simulink model "gm_gauss_sobel_rgb_64bit_full"  (R2022a)
settings: Solver=VariableStepAuto  StartTime=0.0  StopTime=10.0  RelTol=1e-3
undefined symbols (not defined in the file or in its folder): blueMax, blueMin, gray, greenMax, greenMin, redMax, redMin
libraries: hdlsllib x62, visionhdlio x6, visionsources x2
(part 2 of 3)

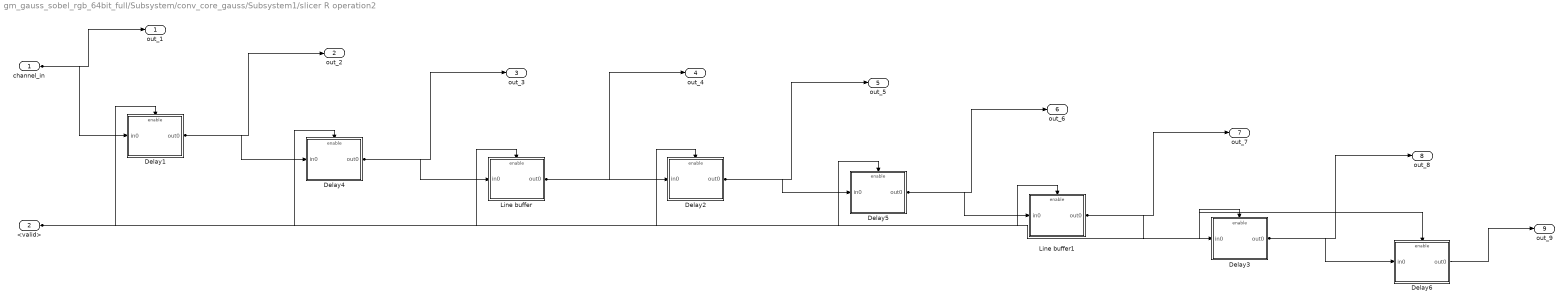
== system gm_gauss_sobel_rgb_64bit_full/Subsystem/conv_core_gauss/Subsystem1/slicer R operation2 ==
  channel_in : Inport  OutDataTypeStr=uint8  PortDimensions=1  SampleTime=2.77039007092199e-06
  <valid> : Inport  Port=2  OutDataTypeStr=boolean  SampleTime=2.77039007092199e-06
  Delay1 : Subsystem
      settings: MinAlgLoopOccurrences=on
  Delay2 : Subsystem
      settings: MinAlgLoopOccurrences=on
  Delay3 : Subsystem
      settings: MinAlgLoopOccurrences=on
  Delay4 : Subsystem
      settings: MinAlgLoopOccurrences=on
  Delay5 : Subsystem
      settings: MinAlgLoopOccurrences=on
  Delay6 : Subsystem
      settings: MinAlgLoopOccurrences=on
  Line buffer : Subsystem
      settings: MinAlgLoopOccurrences=on
  Line buffer1 : Subsystem
      settings: MinAlgLoopOccurrences=on
  out_1 : Outport  SampleTime=2.77039007092199e-06  InitialOutput=0  VectorParamsAs1DForOutWhenUnconnected=off
  out_2 : Outport  Port=2  SampleTime=2.77039007092199e-06  InitialOutput=0  VectorParamsAs1DForOutWhenUnconnected=off
  out_3 : Outport  Port=3  SampleTime=2.77039007092199e-06  InitialOutput=0  VectorParamsAs1DForOutWhenUnconnected=off
  out_4 : Outport  Port=4  SampleTime=2.77039007092199e-06  InitialOutput=0  VectorParamsAs1DForOutWhenUnconnected=off
  out_5 : Outport  Port=5  SampleTime=2.77039007092199e-06  InitialOutput=0  VectorParamsAs1DForOutWhenUnconnected=off
  out_6 : Outport  Port=6  SampleTime=2.77039007092199e-06  InitialOutput=0  VectorParamsAs1DForOutWhenUnconnected=off
  out_7 : Outport  Port=7  SampleTime=2.77039007092199e-06  InitialOutput=0  VectorParamsAs1DForOutWhenUnconnected=off
  out_8 : Outport  Port=8  SampleTime=2.77039007092199e-06  InitialOutput=0  VectorParamsAs1DForOutWhenUnconnected=off
  out_9 : Outport  Port=9  SampleTime=2.77039007092199e-06  InitialOutput=0  VectorParamsAs1DForOutWhenUnconnected=off
  wires:
  channel_in/1 -> Delay1/1(in0), out_1/1
  Delay1/1(out0) -> Delay4/1(in0), out_2/1
  Delay2/1(out0) -> Delay5/1(in0), out_5/1
  Delay3/1(out0) -> Delay6/1(in0), out_8/1
  Delay4/1(out0) -> Line buffer/1(in0), out_3/1
  Delay5/1(out0) -> Line buffer1/1(in0), out_6/1
  Delay6/1(out0) -> out_9/1
  Line buffer/1(out0) -> Delay2/1(in0), out_4/1
  Line buffer1/1(out0) -> Delay3/1(in0), out_7/1
  <valid>/1 -> Line buffer1/Enable, Line buffer/Enable, Delay6/Enable, Delay5/Enable, Delay4/Enable, Delay3/Enable, Delay2/Enable, Delay1/Enable

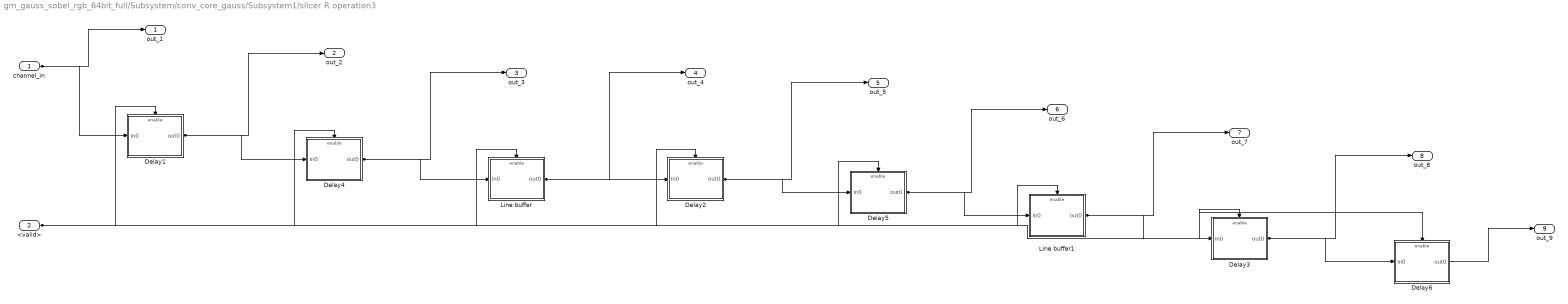
== system gm_gauss_sobel_rgb_64bit_full/Subsystem/conv_core_gauss/Subsystem1/slicer R operation3 ==
  channel_in : Inport  OutDataTypeStr=uint8  PortDimensions=1  SampleTime=2.77039007092199e-06
  <valid> : Inport  Port=2  OutDataTypeStr=boolean  SampleTime=2.77039007092199e-06
  Delay1 : Subsystem
      settings: MinAlgLoopOccurrences=on
  Delay2 : Subsystem
      settings: MinAlgLoopOccurrences=on
  Delay3 : Subsystem
      settings: MinAlgLoopOccurrences=on
  Delay4 : Subsystem
      settings: MinAlgLoopOccurrences=on
  Delay5 : Subsystem
      settings: MinAlgLoopOccurrences=on
  Delay6 : Subsystem
      settings: MinAlgLoopOccurrences=on
  Line buffer : Subsystem
      settings: MinAlgLoopOccurrences=on
  Line buffer1 : Subsystem
      settings: MinAlgLoopOccurrences=on
  out_1 : Outport  SampleTime=2.77039007092199e-06  InitialOutput=0  VectorParamsAs1DForOutWhenUnconnected=off
  out_2 : Outport  Port=2  SampleTime=2.77039007092199e-06  InitialOutput=0  VectorParamsAs1DForOutWhenUnconnected=off
  out_3 : Outport  Port=3  SampleTime=2.77039007092199e-06  InitialOutput=0  VectorParamsAs1DForOutWhenUnconnected=off
  out_4 : Outport  Port=4  SampleTime=2.77039007092199e-06  InitialOutput=0  VectorParamsAs1DForOutWhenUnconnected=off
  out_5 : Outport  Port=5  SampleTime=2.77039007092199e-06  InitialOutput=0  VectorParamsAs1DForOutWhenUnconnected=off
  out_6 : Outport  Port=6  SampleTime=2.77039007092199e-06  InitialOutput=0  VectorParamsAs1DForOutWhenUnconnected=off
  out_7 : Outport  Port=7  SampleTime=2.77039007092199e-06  InitialOutput=0  VectorParamsAs1DForOutWhenUnconnected=off
  out_8 : Outport  Port=8  SampleTime=2.77039007092199e-06  InitialOutput=0  VectorParamsAs1DForOutWhenUnconnected=off
  out_9 : Outport  Port=9  SampleTime=2.77039007092199e-06  InitialOutput=0  VectorParamsAs1DForOutWhenUnconnected=off
  wires:
  channel_in/1 -> Delay1/1(in0), out_1/1
  Delay1/1(out0) -> Delay4/1(in0), out_2/1
  Delay2/1(out0) -> Delay5/1(in0), out_5/1
  Delay3/1(out0) -> Delay6/1(in0), out_8/1
  Delay4/1(out0) -> Line buffer/1(in0), out_3/1
  Delay5/1(out0) -> Line buffer1/1(in0), out_6/1
  Delay6/1(out0) -> out_9/1
  Line buffer/1(out0) -> Delay2/1(in0), out_4/1
  Line buffer1/1(out0) -> Delay3/1(in0), out_7/1
  <valid>/1 -> Line buffer1/Enable, Line buffer/Enable, Delay6/Enable, Delay5/Enable, Delay4/Enable, Delay3/Enable, Delay2/Enable, Delay1/Enable

== system gm_gauss_sobel_rgb_64bit_full/Subsystem/conv_core_gauss/Subsystem1/slicer R operation4 ==
  channel_in : Inport  OutDataTypeStr=uint8  PortDimensions=1  SampleTime=2.77039007092199e-06
  <valid> : Inport  Port=2  OutDataTypeStr=boolean  SampleTime=2.77039007092199e-06
  Delay1 : Subsystem
      settings: MinAlgLoopOccurrences=on
  Delay2 : Subsystem
      settings: MinAlgLoopOccurrences=on
  Delay3 : Subsystem
      settings: MinAlgLoopOccurrences=on
  Delay4 : Subsystem
      settings: MinAlgLoopOccurrences=on
  Delay5 : Subsystem
      settings: MinAlgLoopOccurrences=on
  Delay6 : Subsystem
      settings: MinAlgLoopOccurrences=on
  Line buffer : Subsystem
      settings: MinAlgLoopOccurrences=on
  Line buffer1 : Subsystem
      settings: MinAlgLoopOccurrences=on
  out_1 : Outport  SampleTime=2.77039007092199e-06  InitialOutput=0  VectorParamsAs1DForOutWhenUnconnected=off
  out_2 : Outport  Port=2  SampleTime=2.77039007092199e-06  InitialOutput=0  VectorParamsAs1DForOutWhenUnconnected=off
  out_3 : Outport  Port=3  SampleTime=2.77039007092199e-06  InitialOutput=0  VectorParamsAs1DForOutWhenUnconnected=off
  out_4 : Outport  Port=4  SampleTime=2.77039007092199e-06  InitialOutput=0  VectorParamsAs1DForOutWhenUnconnected=off
  out_5 : Outport  Port=5  SampleTime=2.77039007092199e-06  InitialOutput=0  VectorParamsAs1DForOutWhenUnconnected=off
  out_6 : Outport  Port=6  SampleTime=2.77039007092199e-06  InitialOutput=0  VectorParamsAs1DForOutWhenUnconnected=off
  out_7 : Outport  Port=7  SampleTime=2.77039007092199e-06  InitialOutput=0  VectorParamsAs1DForOutWhenUnconnected=off
  out_8 : Outport  Port=8  SampleTime=2.77039007092199e-06  InitialOutput=0  VectorParamsAs1DForOutWhenUnconnected=off
  out_9 : Outport  Port=9  SampleTime=2.77039007092199e-06  InitialOutput=0  VectorParamsAs1DForOutWhenUnconnected=off
  wires:
  channel_in/1 -> Delay1/1(in0), out_1/1
  Delay1/1(out0) -> Delay4/1(in0), out_2/1
  Delay2/1(out0) -> Delay5/1(in0), out_5/1
  Delay3/1(out0) -> Delay6/1(in0), out_8/1
  Delay4/1(out0) -> Line buffer/1(in0), out_3/1
  Delay5/1(out0) -> Line buffer1/1(in0), out_6/1
  Delay6/1(out0) -> out_9/1
  Line buffer/1(out0) -> Delay2/1(in0), out_4/1
  Line buffer1/1(out0) -> Delay3/1(in0), out_7/1
  <valid>/1 -> Line buffer1/Enable, Line buffer/Enable, Delay6/Enable, Delay5/Enable, Delay4/Enable, Delay3/Enable, Delay2/Enable, Delay1/Enable

== system gm_gauss_sobel_rgb_64bit_full/Subsystem/conv_core_gauss/Subsystem1/slicer R operation5 ==
  channel_in : Inport  OutDataTypeStr=uint8  PortDimensions=1  SampleTime=2.77039007092199e-06
  <valid> : Inport  Port=2  OutDataTypeStr=boolean  SampleTime=2.77039007092199e-06
  Delay1 : Subsystem
      settings: MinAlgLoopOccurrences=on
  Delay2 : Subsystem
      settings: MinAlgLoopOccurrences=on
  Delay3 : Subsystem
      settings: MinAlgLoopOccurrences=on
  Delay4 : Subsystem
      settings: MinAlgLoopOccurrences=on
  Delay5 : Subsystem
      settings: MinAlgLoopOccurrences=on
  Delay6 : Subsystem
      settings: MinAlgLoopOccurrences=on
  Line buffer : Subsystem
      settings: MinAlgLoopOccurrences=on
  Line buffer1 : Subsystem
      settings: MinAlgLoopOccurrences=on
  out_1 : Outport  SampleTime=2.77039007092199e-06  InitialOutput=0  VectorParamsAs1DForOutWhenUnconnected=off
  out_2 : Outport  Port=2  SampleTime=2.77039007092199e-06  InitialOutput=0  VectorParamsAs1DForOutWhenUnconnected=off
  out_3 : Outport  Port=3  SampleTime=2.77039007092199e-06  InitialOutput=0  VectorParamsAs1DForOutWhenUnconnected=off
  out_4 : Outport  Port=4  SampleTime=2.77039007092199e-06  InitialOutput=0  VectorParamsAs1DForOutWhenUnconnected=off
  out_5 : Outport  Port=5  SampleTime=2.77039007092199e-06  InitialOutput=0  VectorParamsAs1DForOutWhenUnconnected=off
  out_6 : Outport  Port=6  SampleTime=2.77039007092199e-06  InitialOutput=0  VectorParamsAs1DForOutWhenUnconnected=off
  out_7 : Outport  Port=7  SampleTime=2.77039007092199e-06  InitialOutput=0  VectorParamsAs1DForOutWhenUnconnected=off
  out_8 : Outport  Port=8  SampleTime=2.77039007092199e-06  InitialOutput=0  VectorParamsAs1DForOutWhenUnconnected=off
  out_9 : Outport  Port=9  SampleTime=2.77039007092199e-06  InitialOutput=0  VectorParamsAs1DForOutWhenUnconnected=off
  wires:
  channel_in/1 -> Delay1/1(in0), out_1/1
  Delay1/1(out0) -> Delay4/1(in0), out_2/1
  Delay2/1(out0) -> Delay5/1(in0), out_5/1
  Delay3/1(out0) -> Delay6/1(in0), out_8/1
  Delay4/1(out0) -> Line buffer/1(in0), out_3/1
  Delay5/1(out0) -> Line buffer1/1(in0), out_6/1
  Delay6/1(out0) -> out_9/1
  Line buffer/1(out0) -> Delay2/1(in0), out_4/1
  Line buffer1/1(out0) -> Delay3/1(in0), out_7/1
  <valid>/1 -> Line buffer1/Enable, Line buffer/Enable, Delay6/Enable, Delay5/Enable, Delay4/Enable, Delay3/Enable, Delay2/Enable, Delay1/Enable

== system gm_gauss_sobel_rgb_64bit_full/Subsystem/conv_core_gauss/Subsystem1/slicer R operation6 ==
  channel_in : Inport  OutDataTypeStr=uint8  PortDimensions=1  SampleTime=2.77039007092199e-06
  <valid> : Inport  Port=2  OutDataTypeStr=boolean  SampleTime=2.77039007092199e-06
  Delay1 : Subsystem
      settings: MinAlgLoopOccurrences=on
  Delay2 : Subsystem
      settings: MinAlgLoopOccurrences=on
  Delay3 : Subsystem
      settings: MinAlgLoopOccurrences=on
  Delay4 : Subsystem
      settings: MinAlgLoopOccurrences=on
  Delay5 : Subsystem
      settings: MinAlgLoopOccurrences=on
  Delay6 : Subsystem
      settings: MinAlgLoopOccurrences=on
  Line buffer : Subsystem
      settings: MinAlgLoopOccurrences=on
  Line buffer1 : Subsystem
      settings: MinAlgLoopOccurrences=on
  out_1 : Outport  SampleTime=2.77039007092199e-06  InitialOutput=0  VectorParamsAs1DForOutWhenUnconnected=off
  out_2 : Outport  Port=2  SampleTime=2.77039007092199e-06  InitialOutput=0  VectorParamsAs1DForOutWhenUnconnected=off
  out_3 : Outport  Port=3  SampleTime=2.77039007092199e-06  InitialOutput=0  VectorParamsAs1DForOutWhenUnconnected=off
  out_4 : Outport  Port=4  SampleTime=2.77039007092199e-06  InitialOutput=0  VectorParamsAs1DForOutWhenUnconnected=off
  out_5 : Outport  Port=5  SampleTime=2.77039007092199e-06  InitialOutput=0  VectorParamsAs1DForOutWhenUnconnected=off
  out_6 : Outport  Port=6  SampleTime=2.77039007092199e-06  InitialOutput=0  VectorParamsAs1DForOutWhenUnconnected=off
  out_7 : Outport  Port=7  SampleTime=2.77039007092199e-06  InitialOutput=0  VectorParamsAs1DForOutWhenUnconnected=off
  out_8 : Outport  Port=8  SampleTime=2.77039007092199e-06  InitialOutput=0  VectorParamsAs1DForOutWhenUnconnected=off
  out_9 : Outport  Port=9  SampleTime=2.77039007092199e-06  InitialOutput=0  VectorParamsAs1DForOutWhenUnconnected=off
  wires:
  channel_in/1 -> Delay1/1(in0), out_1/1
  Delay1/1(out0) -> Delay4/1(in0), out_2/1
  Delay2/1(out0) -> Delay5/1(in0), out_5/1
  Delay3/1(out0) -> Delay6/1(in0), out_8/1
  Delay4/1(out0) -> Line buffer/1(in0), out_3/1
  Delay5/1(out0) -> Line buffer1/1(in0), out_6/1
  Delay6/1(out0) -> out_9/1
  Line buffer/1(out0) -> Delay2/1(in0), out_4/1
  Line buffer1/1(out0) -> Delay3/1(in0), out_7/1
  <valid>/1 -> Line buffer1/Enable, Line buffer/Enable, Delay6/Enable, Delay5/Enable, Delay4/Enable, Delay3/Enable, Delay2/Enable, Delay1/Enable

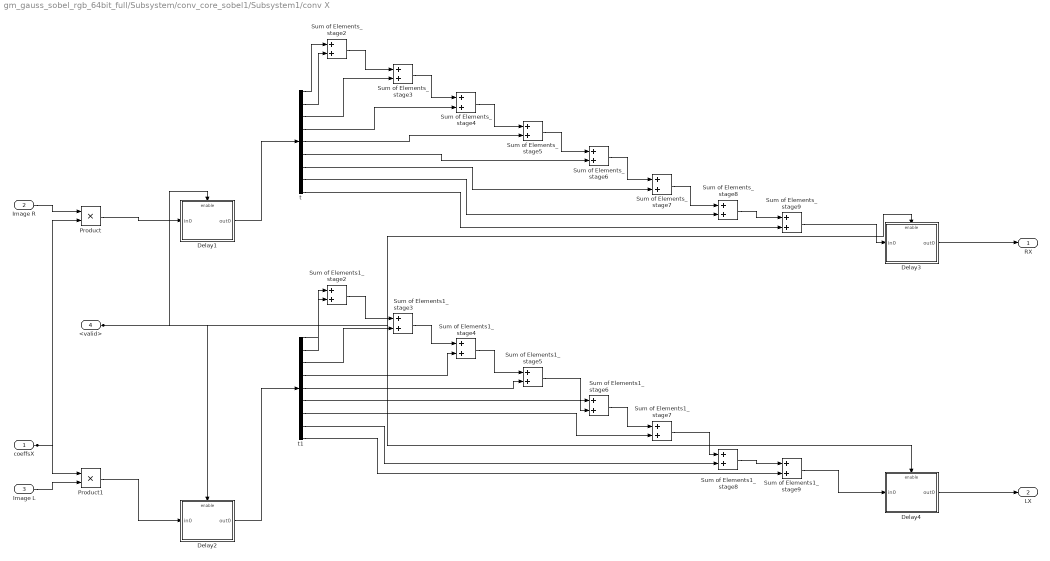
== system gm_gauss_sobel_rgb_64bit_full/Subsystem/conv_core_sobel1/Subsystem1/conv X ==
  coeffsX : Inport  OutDataTypeStr=int8  PortDimensions=[9]  SampleTime=2.77039007092199e-06
  Image R : Inport  Port=2  OutDataTypeStr=uint8  PortDimensions=[9]  SampleTime=2.77039007092199e-06
  Image L : Inport  Port=3  OutDataTypeStr=uint8  PortDimensions=[9]  SampleTime=2.77039007092199e-06
  <valid> : Inport  Port=4  OutDataTypeStr=boolean  SampleTime=2.77039007092199e-06
  Delay1 : Subsystem
      settings: MinAlgLoopOccurrences=on
  Delay2 : Subsystem
      settings: MinAlgLoopOccurrences=on
  Delay3 : Subsystem
      settings: MinAlgLoopOccurrences=on
  Delay4 : Subsystem
      settings: MinAlgLoopOccurrences=on
  Product : Product  Inputs=**  OutDataTypeStr=int16  SaturateOnIntegerOverflow=on  SampleTime=2.77039007092199e-06
  Product1 : Product  Inputs=**  OutDataTypeStr=int16  SaturateOnIntegerOverflow=on  SampleTime=2.77039007092199e-06
  Sum of Elements1_stage{2..8} (7 alike) : Sum  AccumDataTypeStr=int32  OutDataTypeStr=int32  SaturateOnIntegerOverflow=on  SampleTime=2.77039007092199e-06
  Sum of Elements1_stage9 : Sum  AccumDataTypeStr=int32  OutDataTypeStr=uint8  SaturateOnIntegerOverflow=on  SampleTime=2.77039007092199e-06
  Sum of Elements_stage{2..8} (7 alike) : Sum  AccumDataTypeStr=int32  OutDataTypeStr=int32  SaturateOnIntegerOverflow=on  SampleTime=2.77039007092199e-06
  Sum of Elements_stage9 : Sum  AccumDataTypeStr=int32  OutDataTypeStr=uint8  SaturateOnIntegerOverflow=on  SampleTime=2.77039007092199e-06
  t : Demux  Outputs=9
  t1 : Demux  Outputs=9
  RX : Outport  SampleTime=2.77039007092199e-06  InitialOutput=0
  LX : Outport  Port=2  SampleTime=2.77039007092199e-06  InitialOutput=0
  wires:
  coeffsX/1 -> Product1/1, Product/2
  Image R/1 -> Product/1
  Image L/1 -> Product1/2
  Delay1/1(out0) -> t/1
  Delay2/1(out0) -> t1/1
  Delay3/1(out0) -> RX/1
  Delay4/1(out0) -> LX/1
  Product/1 -> Delay1/1(in0)
  Product1/1 -> Delay2/1(in0)
  <valid>/1 -> Delay4/Enable, Delay3/Enable, Delay2/Enable, Delay1/Enable
  Sum of Elements_stage9/1 -> Delay3/1(in0)
  t/1 -> Sum of Elements_stage2/1
  t/2 -> Sum of Elements_stage2/2
  t/3 -> Sum of Elements_stage3/2
  t/4 -> Sum of Elements_stage4/2
  t/5 -> Sum of Elements_stage5/2
  t/6 -> Sum of Elements_stage6/2
  t/7 -> Sum of Elements_stage7/2
  t/8 -> Sum of Elements_stage8/2
  t/9 -> Sum of Elements_stage9/2
  Sum of Elements_stage2/1 -> Sum of Elements_stage3/1
  Sum of Elements_stage3/1 -> Sum of Elements_stage4/1
  Sum of Elements_stage4/1 -> Sum of Elements_stage5/1
  Sum of Elements_stage5/1 -> Sum of Elements_stage6/1
  Sum of Elements_stage6/1 -> Sum of Elements_stage7/1
  Sum of Elements_stage7/1 -> Sum of Elements_stage8/1
  Sum of Elements_stage8/1 -> Sum of Elements_stage9/1
  Sum of Elements1_stage9/1 -> Delay4/1(in0)
  t1/1 -> Sum of Elements1_stage2/1
  t1/2 -> Sum of Elements1_stage2/2
  t1/3 -> Sum of Elements1_stage3/2
  t1/4 -> Sum of Elements1_stage4/2
  t1/5 -> Sum of Elements1_stage5/2
  t1/6 -> Sum of Elements1_stage6/2
  t1/7 -> Sum of Elements1_stage7/2
  t1/8 -> Sum of Elements1_stage8/2
  t1/9 -> Sum of Elements1_stage9/2
  Sum of Elements1_stage2/1 -> Sum of Elements1_stage3/1
  Sum of Elements1_stage3/1 -> Sum of Elements1_stage4/1
  Sum of Elements1_stage4/1 -> Sum of Elements1_stage5/1
  Sum of Elements1_stage5/1 -> Sum of Elements1_stage6/1
  Sum of Elements1_stage6/1 -> Sum of Elements1_stage7/1
  Sum of Elements1_stage7/1 -> Sum of Elements1_stage8/1
  Sum of Elements1_stage8/1 -> Sum of Elements1_stage9/1

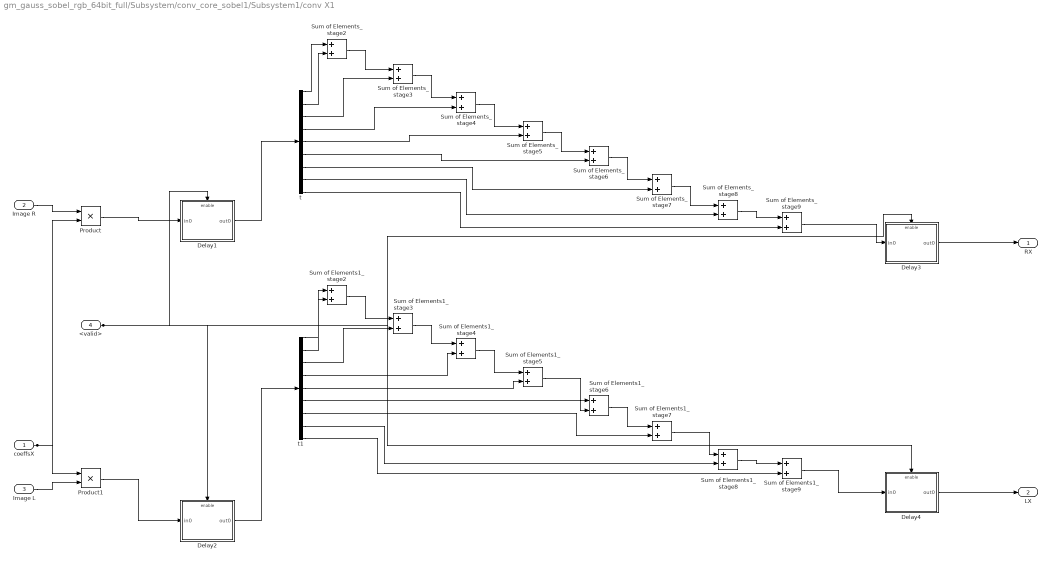
== system gm_gauss_sobel_rgb_64bit_full/Subsystem/conv_core_sobel1/Subsystem1/conv X1 ==
  coeffsX : Inport  OutDataTypeStr=int8  PortDimensions=[9]  SampleTime=2.77039007092199e-06
  Image R : Inport  Port=2  OutDataTypeStr=uint8  PortDimensions=[9]  SampleTime=2.77039007092199e-06
  Image L : Inport  Port=3  OutDataTypeStr=uint8  PortDimensions=[9]  SampleTime=2.77039007092199e-06
  <valid> : Inport  Port=4  OutDataTypeStr=boolean  SampleTime=2.77039007092199e-06
  Delay1 : Subsystem
      settings: MinAlgLoopOccurrences=on
  Delay2 : Subsystem
      settings: MinAlgLoopOccurrences=on
  Delay3 : Subsystem
      settings: MinAlgLoopOccurrences=on
  Delay4 : Subsystem
      settings: MinAlgLoopOccurrences=on
  Product : Product  Inputs=**  OutDataTypeStr=int16  SaturateOnIntegerOverflow=on  SampleTime=2.77039007092199e-06
  Product1 : Product  Inputs=**  OutDataTypeStr=int16  SaturateOnIntegerOverflow=on  SampleTime=2.77039007092199e-06
  Sum of Elements1_stage{2..8} (7 alike) : Sum  AccumDataTypeStr=int32  OutDataTypeStr=int32  SaturateOnIntegerOverflow=on  SampleTime=2.77039007092199e-06
  Sum of Elements1_stage9 : Sum  AccumDataTypeStr=int32  OutDataTypeStr=uint8  SaturateOnIntegerOverflow=on  SampleTime=2.77039007092199e-06
  Sum of Elements_stage{2..8} (7 alike) : Sum  AccumDataTypeStr=int32  OutDataTypeStr=int32  SaturateOnIntegerOverflow=on  SampleTime=2.77039007092199e-06
  Sum of Elements_stage9 : Sum  AccumDataTypeStr=int32  OutDataTypeStr=uint8  SaturateOnIntegerOverflow=on  SampleTime=2.77039007092199e-06
  t : Demux  Outputs=9
  t1 : Demux  Outputs=9
  RX : Outport  SampleTime=2.77039007092199e-06  InitialOutput=0
  LX : Outport  Port=2  SampleTime=2.77039007092199e-06  InitialOutput=0
  wires:
  coeffsX/1 -> Product1/1, Product/2
  Image R/1 -> Product/1
  Image L/1 -> Product1/2
  Delay1/1(out0) -> t/1
  Delay2/1(out0) -> t1/1
  Delay3/1(out0) -> RX/1
  Delay4/1(out0) -> LX/1
  Product/1 -> Delay1/1(in0)
  Product1/1 -> Delay2/1(in0)
  <valid>/1 -> Delay4/Enable, Delay3/Enable, Delay2/Enable, Delay1/Enable
  Sum of Elements_stage9/1 -> Delay3/1(in0)
  t/1 -> Sum of Elements_stage2/1
  t/2 -> Sum of Elements_stage2/2
  t/3 -> Sum of Elements_stage3/2
  t/4 -> Sum of Elements_stage4/2
  t/5 -> Sum of Elements_stage5/2
  t/6 -> Sum of Elements_stage6/2
  t/7 -> Sum of Elements_stage7/2
  t/8 -> Sum of Elements_stage8/2
  t/9 -> Sum of Elements_stage9/2
  Sum of Elements_stage2/1 -> Sum of Elements_stage3/1
  Sum of Elements_stage3/1 -> Sum of Elements_stage4/1
  Sum of Elements_stage4/1 -> Sum of Elements_stage5/1
  Sum of Elements_stage5/1 -> Sum of Elements_stage6/1
  Sum of Elements_stage6/1 -> Sum of Elements_stage7/1
  Sum of Elements_stage7/1 -> Sum of Elements_stage8/1
  Sum of Elements_stage8/1 -> Sum of Elements_stage9/1
  Sum of Elements1_stage9/1 -> Delay4/1(in0)
  t1/1 -> Sum of Elements1_stage2/1
  t1/2 -> Sum of Elements1_stage2/2
  t1/3 -> Sum of Elements1_stage3/2
  t1/4 -> Sum of Elements1_stage4/2
  t1/5 -> Sum of Elements1_stage5/2
  t1/6 -> Sum of Elements1_stage6/2
  t1/7 -> Sum of Elements1_stage7/2
  t1/8 -> Sum of Elements1_stage8/2
  t1/9 -> Sum of Elements1_stage9/2
  Sum of Elements1_stage2/1 -> Sum of Elements1_stage3/1
  Sum of Elements1_stage3/1 -> Sum of Elements1_stage4/1
  Sum of Elements1_stage4/1 -> Sum of Elements1_stage5/1
  Sum of Elements1_stage5/1 -> Sum of Elements1_stage6/1
  Sum of Elements1_stage6/1 -> Sum of Elements1_stage7/1
  Sum of Elements1_stage7/1 -> Sum of Elements1_stage8/1
  Sum of Elements1_stage8/1 -> Sum of Elements1_stage9/1

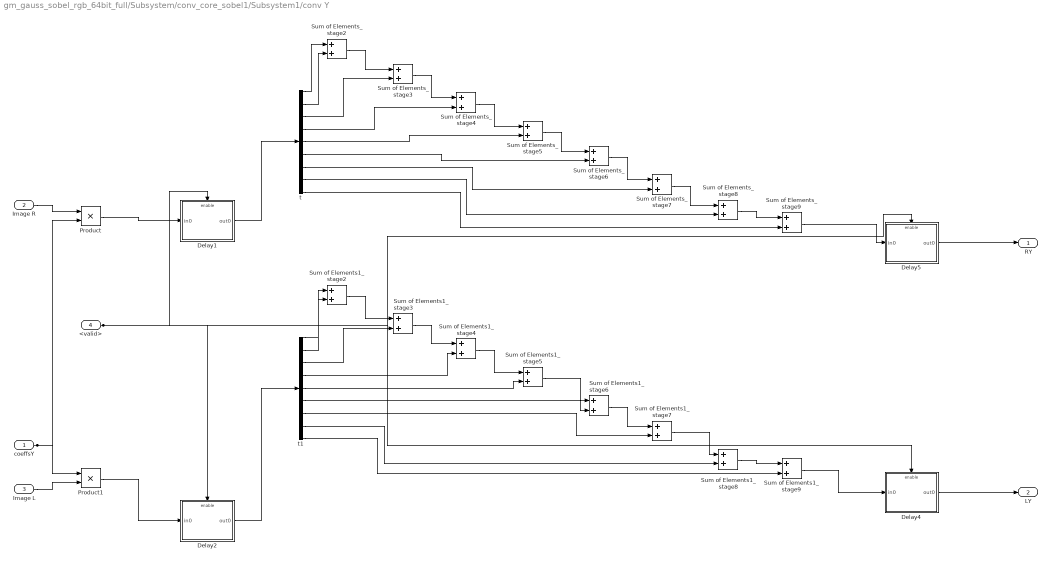
== system gm_gauss_sobel_rgb_64bit_full/Subsystem/conv_core_sobel1/Subsystem1/conv Y ==
  coeffsY : Inport  OutDataTypeStr=int8  PortDimensions=[9]  SampleTime=2.77039007092199e-06
  Image R : Inport  Port=2  OutDataTypeStr=uint8  PortDimensions=[9]  SampleTime=2.77039007092199e-06
  Image L : Inport  Port=3  OutDataTypeStr=uint8  PortDimensions=[9]  SampleTime=2.77039007092199e-06
  <valid> : Inport  Port=4  OutDataTypeStr=boolean  SampleTime=2.77039007092199e-06
  Delay1 : Subsystem
      settings: MinAlgLoopOccurrences=on
  Delay2 : Subsystem
      settings: MinAlgLoopOccurrences=on
  Delay4 : Subsystem
      settings: MinAlgLoopOccurrences=on
  Delay5 : Subsystem
      settings: MinAlgLoopOccurrences=on
  Product : Product  Inputs=**  OutDataTypeStr=int16  SaturateOnIntegerOverflow=on  SampleTime=2.77039007092199e-06
  Product1 : Product  Inputs=**  OutDataTypeStr=int16  SaturateOnIntegerOverflow=on  SampleTime=2.77039007092199e-06
  Sum of Elements1_stage{2..8} (7 alike) : Sum  AccumDataTypeStr=int32  OutDataTypeStr=int32  SaturateOnIntegerOverflow=on  SampleTime=2.77039007092199e-06
  Sum of Elements1_stage9 : Sum  AccumDataTypeStr=int32  OutDataTypeStr=uint8  SaturateOnIntegerOverflow=on  SampleTime=2.77039007092199e-06
  Sum of Elements_stage{2..8} (7 alike) : Sum  AccumDataTypeStr=int32  OutDataTypeStr=int32  SaturateOnIntegerOverflow=on  SampleTime=2.77039007092199e-06
  Sum of Elements_stage9 : Sum  AccumDataTypeStr=int32  OutDataTypeStr=uint8  SaturateOnIntegerOverflow=on  SampleTime=2.77039007092199e-06
  t : Demux  Outputs=9
  t1 : Demux  Outputs=9
  RY : Outport  SampleTime=2.77039007092199e-06  InitialOutput=0
  LY : Outport  Port=2  SampleTime=2.77039007092199e-06  InitialOutput=0
  wires:
  coeffsY/1 -> Product1/1, Product/2
  Image R/1 -> Product/1
  Image L/1 -> Product1/2
  Delay1/1(out0) -> t/1
  Delay2/1(out0) -> t1/1
  Delay4/1(out0) -> LY/1
  Delay5/1(out0) -> RY/1
  Product/1 -> Delay1/1(in0)
  Product1/1 -> Delay2/1(in0)
  <valid>/1 -> Delay5/Enable, Delay4/Enable, Delay2/Enable, Delay1/Enable
  Sum of Elements_stage9/1 -> Delay5/1(in0)
  t/1 -> Sum of Elements_stage2/1
  t/2 -> Sum of Elements_stage2/2
  t/3 -> Sum of Elements_stage3/2
  t/4 -> Sum of Elements_stage4/2
  t/5 -> Sum of Elements_stage5/2
  t/6 -> Sum of Elements_stage6/2
  t/7 -> Sum of Elements_stage7/2
  t/8 -> Sum of Elements_stage8/2
  t/9 -> Sum of Elements_stage9/2
  Sum of Elements_stage2/1 -> Sum of Elements_stage3/1
  Sum of Elements_stage3/1 -> Sum of Elements_stage4/1
  Sum of Elements_stage4/1 -> Sum of Elements_stage5/1
  Sum of Elements_stage5/1 -> Sum of Elements_stage6/1
  Sum of Elements_stage6/1 -> Sum of Elements_stage7/1
  Sum of Elements_stage7/1 -> Sum of Elements_stage8/1
  Sum of Elements_stage8/1 -> Sum of Elements_stage9/1
  Sum of Elements1_stage9/1 -> Delay4/1(in0)
  t1/1 -> Sum of Elements1_stage2/1
  t1/2 -> Sum of Elements1_stage2/2
  t1/3 -> Sum of Elements1_stage3/2
  t1/4 -> Sum of Elements1_stage4/2
  t1/5 -> Sum of Elements1_stage5/2
  t1/6 -> Sum of Elements1_stage6/2
  t1/7 -> Sum of Elements1_stage7/2
  t1/8 -> Sum of Elements1_stage8/2
  t1/9 -> Sum of Elements1_stage9/2
  Sum of Elements1_stage2/1 -> Sum of Elements1_stage3/1
  Sum of Elements1_stage3/1 -> Sum of Elements1_stage4/1
  Sum of Elements1_stage4/1 -> Sum of Elements1_stage5/1
  Sum of Elements1_stage5/1 -> Sum of Elements1_stage6/1
  Sum of Elements1_stage6/1 -> Sum of Elements1_stage7/1
  Sum of Elements1_stage7/1 -> Sum of Elements1_stage8/1
  Sum of Elements1_stage8/1 -> Sum of Elements1_stage9/1

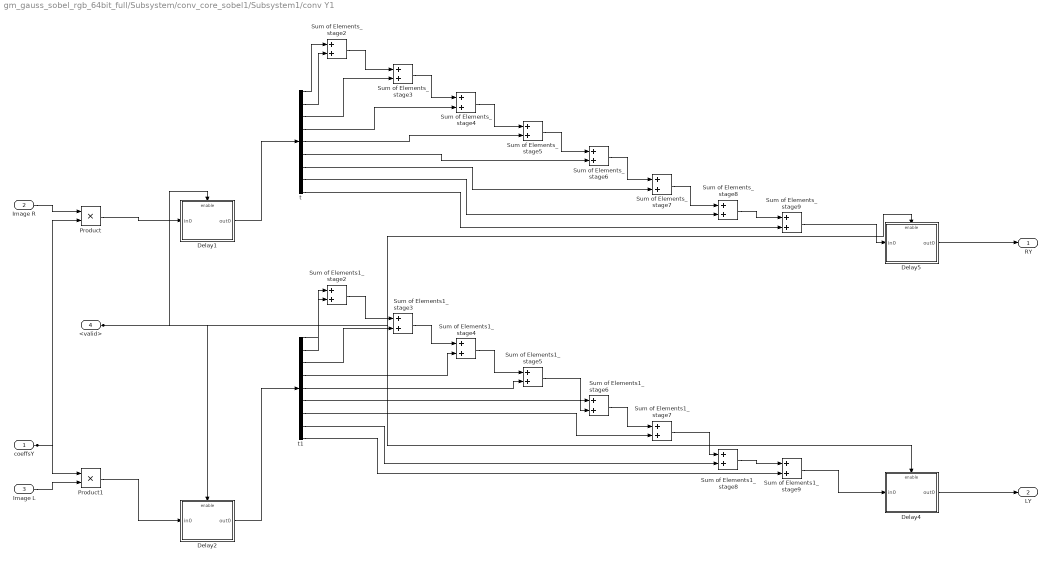
== system gm_gauss_sobel_rgb_64bit_full/Subsystem/conv_core_sobel1/Subsystem1/conv Y1 ==
  coeffsY : Inport  OutDataTypeStr=int8  PortDimensions=[9]  SampleTime=2.77039007092199e-06
  Image R : Inport  Port=2  OutDataTypeStr=uint8  PortDimensions=[9]  SampleTime=2.77039007092199e-06
  Image L : Inport  Port=3  OutDataTypeStr=uint8  PortDimensions=[9]  SampleTime=2.77039007092199e-06
  <valid> : Inport  Port=4  OutDataTypeStr=boolean  SampleTime=2.77039007092199e-06
  Delay1 : Subsystem
      settings: MinAlgLoopOccurrences=on
  Delay2 : Subsystem
      settings: MinAlgLoopOccurrences=on
  Delay4 : Subsystem
      settings: MinAlgLoopOccurrences=on
  Delay5 : Subsystem
      settings: MinAlgLoopOccurrences=on
  Product : Product  Inputs=**  OutDataTypeStr=int16  SaturateOnIntegerOverflow=on  SampleTime=2.77039007092199e-06
  Product1 : Product  Inputs=**  OutDataTypeStr=int16  SaturateOnIntegerOverflow=on  SampleTime=2.77039007092199e-06
  Sum of Elements1_stage{2..8} (7 alike) : Sum  AccumDataTypeStr=int32  OutDataTypeStr=int32  SaturateOnIntegerOverflow=on  SampleTime=2.77039007092199e-06
  Sum of Elements1_stage9 : Sum  AccumDataTypeStr=int32  OutDataTypeStr=uint8  SaturateOnIntegerOverflow=on  SampleTime=2.77039007092199e-06
  Sum of Elements_stage{2..8} (7 alike) : Sum  AccumDataTypeStr=int32  OutDataTypeStr=int32  SaturateOnIntegerOverflow=on  SampleTime=2.77039007092199e-06
  Sum of Elements_stage9 : Sum  AccumDataTypeStr=int32  OutDataTypeStr=uint8  SaturateOnIntegerOverflow=on  SampleTime=2.77039007092199e-06
  t : Demux  Outputs=9
  t1 : Demux  Outputs=9
  RY : Outport  SampleTime=2.77039007092199e-06  InitialOutput=0
  LY : Outport  Port=2  SampleTime=2.77039007092199e-06  InitialOutput=0
  wires:
  coeffsY/1 -> Product1/1, Product/2
  Image R/1 -> Product/1
  Image L/1 -> Product1/2
  Delay1/1(out0) -> t/1
  Delay2/1(out0) -> t1/1
  Delay4/1(out0) -> LY/1
  Delay5/1(out0) -> RY/1
  Product/1 -> Delay1/1(in0)
  Product1/1 -> Delay2/1(in0)
  <valid>/1 -> Delay5/Enable, Delay4/Enable, Delay2/Enable, Delay1/Enable
  Sum of Elements_stage9/1 -> Delay5/1(in0)
  t/1 -> Sum of Elements_stage2/1
  t/2 -> Sum of Elements_stage2/2
  t/3 -> Sum of Elements_stage3/2
  t/4 -> Sum of Elements_stage4/2
  t/5 -> Sum of Elements_stage5/2
  t/6 -> Sum of Elements_stage6/2
  t/7 -> Sum of Elements_stage7/2
  t/8 -> Sum of Elements_stage8/2
  t/9 -> Sum of Elements_stage9/2
  Sum of Elements_stage2/1 -> Sum of Elements_stage3/1
  Sum of Elements_stage3/1 -> Sum of Elements_stage4/1
  Sum of Elements_stage4/1 -> Sum of Elements_stage5/1
  Sum of Elements_stage5/1 -> Sum of Elements_stage6/1
  Sum of Elements_stage6/1 -> Sum of Elements_stage7/1
  Sum of Elements_stage7/1 -> Sum of Elements_stage8/1
  Sum of Elements_stage8/1 -> Sum of Elements_stage9/1
  Sum of Elements1_stage9/1 -> Delay4/1(in0)
  t1/1 -> Sum of Elements1_stage2/1
  t1/2 -> Sum of Elements1_stage2/2
  t1/3 -> Sum of Elements1_stage3/2
  t1/4 -> Sum of Elements1_stage4/2
  t1/5 -> Sum of Elements1_stage5/2
  t1/6 -> Sum of Elements1_stage6/2
  t1/7 -> Sum of Elements1_stage7/2
  t1/8 -> Sum of Elements1_stage8/2
  t1/9 -> Sum of Elements1_stage9/2
  Sum of Elements1_stage2/1 -> Sum of Elements1_stage3/1
  Sum of Elements1_stage3/1 -> Sum of Elements1_stage4/1
  Sum of Elements1_stage4/1 -> Sum of Elements1_stage5/1
  Sum of Elements1_stage5/1 -> Sum of Elements1_stage6/1
  Sum of Elements1_stage6/1 -> Sum of Elements1_stage7/1
  Sum of Elements1_stage7/1 -> Sum of Elements1_stage8/1
  Sum of Elements1_stage8/1 -> Sum of Elements1_stage9/1

== system gm_gauss_sobel_rgb_64bit_full/Subsystem/conv_core_sobel1/Subsystem1/slicer L operation1 ==
  channel_in : Inport  OutDataTypeStr=uint8  PortDimensions=1  SampleTime=2.77039007092199e-06
  <valid> : Inport  Port=2  OutDataTypeStr=boolean  SampleTime=2.77039007092199e-06
  Delay1 : Subsystem
      settings: MinAlgLoopOccurrences=on
  Delay2 : Subsystem
      settings: MinAlgLoopOccurrences=on
  Delay3 : Subsystem
      settings: MinAlgLoopOccurrences=on
  Delay4 : Subsystem
      settings: MinAlgLoopOccurrences=on
  Delay5 : Subsystem
      settings: MinAlgLoopOccurrences=on
  Delay6 : Subsystem
      settings: MinAlgLoopOccurrences=on
  Line buffer : Subsystem
      settings: MinAlgLoopOccurrences=on
  Line buffer1 : Subsystem
      settings: MinAlgLoopOccurrences=on
  out_1 : Outport  SampleTime=2.77039007092199e-06  InitialOutput=0  VectorParamsAs1DForOutWhenUnconnected=off
  out_2 : Outport  Port=2  SampleTime=2.77039007092199e-06  InitialOutput=0  VectorParamsAs1DForOutWhenUnconnected=off
  out_3 : Outport  Port=3  SampleTime=2.77039007092199e-06  InitialOutput=0  VectorParamsAs1DForOutWhenUnconnected=off
  out_4 : Outport  Port=4  SampleTime=2.77039007092199e-06  InitialOutput=0  VectorParamsAs1DForOutWhenUnconnected=off
  out_5 : Outport  Port=5  SampleTime=2.77039007092199e-06  InitialOutput=0  VectorParamsAs1DForOutWhenUnconnected=off
  out_6 : Outport  Port=6  SampleTime=2.77039007092199e-06  InitialOutput=0  VectorParamsAs1DForOutWhenUnconnected=off
  out_7 : Outport  Port=7  SampleTime=2.77039007092199e-06  InitialOutput=0  VectorParamsAs1DForOutWhenUnconnected=off
  out_8 : Outport  Port=8  SampleTime=2.77039007092199e-06  InitialOutput=0  VectorParamsAs1DForOutWhenUnconnected=off
  out_9 : Outport  Port=9  SampleTime=2.77039007092199e-06  InitialOutput=0  VectorParamsAs1DForOutWhenUnconnected=off
  wires:
  channel_in/1 -> Delay1/1(in0), out_1/1
  Delay1/1(out0) -> Delay4/1(in0), out_2/1
  Delay2/1(out0) -> Delay5/1(in0), out_5/1
  Delay3/1(out0) -> Delay6/1(in0), out_8/1
  Delay4/1(out0) -> Line buffer/1(in0), out_3/1
  Delay5/1(out0) -> Line buffer1/1(in0), out_6/1
  Delay6/1(out0) -> out_9/1
  Line buffer/1(out0) -> Delay2/1(in0), out_4/1
  Line buffer1/1(out0) -> Delay3/1(in0), out_7/1
  <valid>/1 -> Line buffer1/Enable, Line buffer/Enable, Delay6/Enable, Delay5/Enable, Delay4/Enable, Delay3/Enable, Delay2/Enable, Delay1/Enable

== system gm_gauss_sobel_rgb_64bit_full/Subsystem/conv_core_sobel1/Subsystem1/slicer R operation ==
  channel_in : Inport  OutDataTypeStr=uint8  PortDimensions=1  SampleTime=2.77039007092199e-06
  <valid> : Inport  Port=2  OutDataTypeStr=boolean  SampleTime=2.77039007092199e-06
  Delay1 : Subsystem
      settings: MinAlgLoopOccurrences=on
  Delay2 : Subsystem
      settings: MinAlgLoopOccurrences=on
  Delay3 : Subsystem
      settings: MinAlgLoopOccurrences=on
  Delay4 : Subsystem
      settings: MinAlgLoopOccurrences=on
  Delay5 : Subsystem
      settings: MinAlgLoopOccurrences=on
  Delay6 : Subsystem
      settings: MinAlgLoopOccurrences=on
  Line buffer : Subsystem
      settings: MinAlgLoopOccurrences=on
  Line buffer1 : Subsystem
      settings: MinAlgLoopOccurrences=on
  out_1 : Outport  SampleTime=2.77039007092199e-06  InitialOutput=0  VectorParamsAs1DForOutWhenUnconnected=off
  out_2 : Outport  Port=2  SampleTime=2.77039007092199e-06  InitialOutput=0  VectorParamsAs1DForOutWhenUnconnected=off
  out_3 : Outport  Port=3  SampleTime=2.77039007092199e-06  InitialOutput=0  VectorParamsAs1DForOutWhenUnconnected=off
  out_4 : Outport  Port=4  SampleTime=2.77039007092199e-06  InitialOutput=0  VectorParamsAs1DForOutWhenUnconnected=off
  out_5 : Outport  Port=5  SampleTime=2.77039007092199e-06  InitialOutput=0  VectorParamsAs1DForOutWhenUnconnected=off
  out_6 : Outport  Port=6  SampleTime=2.77039007092199e-06  InitialOutput=0  VectorParamsAs1DForOutWhenUnconnected=off
  out_7 : Outport  Port=7  SampleTime=2.77039007092199e-06  InitialOutput=0  VectorParamsAs1DForOutWhenUnconnected=off
  out_8 : Outport  Port=8  SampleTime=2.77039007092199e-06  InitialOutput=0  VectorParamsAs1DForOutWhenUnconnected=off
  out_9 : Outport  Port=9  SampleTime=2.77039007092199e-06  InitialOutput=0  VectorParamsAs1DForOutWhenUnconnected=off
  wires:
  channel_in/1 -> Delay1/1(in0), out_1/1
  Delay1/1(out0) -> Delay4/1(in0), out_2/1
  Delay2/1(out0) -> Delay5/1(in0), out_5/1
  Delay3/1(out0) -> Delay6/1(in0), out_8/1
  Delay4/1(out0) -> Line buffer/1(in0), out_3/1
  Delay5/1(out0) -> Line buffer1/1(in0), out_6/1
  Delay6/1(out0) -> out_9/1
  Line buffer/1(out0) -> Delay2/1(in0), out_4/1
  Line buffer1/1(out0) -> Delay3/1(in0), out_7/1
  <valid>/1 -> Line buffer1/Enable, Line buffer/Enable, Delay6/Enable, Delay5/Enable, Delay4/Enable, Delay3/Enable, Delay2/Enable, Delay1/Enable

== system gm_gauss_sobel_rgb_64bit_full/Subsystem/rgb_filter/Subsystem1/Delay1 ==
  in0 : Inport  OutDataTypeStr=fixdt(0,32,0,'DataTypeOverride', 'Off')  SampleTime=2.77039007092199e-06
  <valid> : EnablePort  OutDataTypeStr=boolean
  Delay1 : Delay  DelayLength=double(1)  InitialCondition=0
  out0 : Outport  OutDataTypeStr=uint32  SampleTime=2.77039007092199e-06  InitialOutput=0
  wires:
  Delay1/1 -> out0/1
  in0/1 -> Delay1/1

== system gm_gauss_sobel_rgb_64bit_full/Subsystem/rgb_filter/Subsystem1/Delay2 ==
  in0 : Inport  OutDataTypeStr=fixdt(0,32,0,'DataTypeOverride', 'Off')  SampleTime=2.77039007092199e-06
  <valid> : EnablePort  OutDataTypeStr=boolean
  Delay2 : Delay  DelayLength=double(1)  InitialCondition=0
  out0 : Outport  OutDataTypeStr=uint32  SampleTime=2.77039007092199e-06  InitialOutput=0
  wires:
  Delay2/1 -> out0/1
  in0/1 -> Delay2/1

== system gm_gauss_sobel_rgb_64bit_full/Subsystem/rgb_filter/Subsystem1/comparison ==
  In1 : Inport  OutDataTypeStr=uint8  PortDimensions=1  SampleTime=2.77039007092199e-06
  max : Inport  Port=2  OutDataTypeStr=uint8  PortDimensions=1  SampleTime=2.77039007092199e-06
  min : Inport  Port=3  OutDataTypeStr=uint8  PortDimensions=1  SampleTime=2.77039007092199e-06
  AND : Logic  IconShape=distinctive  AllPortsSameDT=off  OutDataTypeStr=boolean
  Constant : Constant  Value=0  OutDataTypeStr=uint8  SampleTime=-1
  Relational Operator : RelationalOperator  Operator=<=  OutDataTypeStr=boolean  RndMeth=Simplest  InputSameDT=off
  Relational Operator1 : RelationalOperator  OutDataTypeStr=boolean  RndMeth=Simplest  InputSameDT=off
  Switch : Switch  Criteria=u2 ~= 0  SaturateOnIntegerOverflow=off  InputSameDT=off
  Out1 : Outport  SampleTime=2.77039007092199e-06  InitialOutput=0
  wires:
  In1/1 -> Switch/1, Relational Operator1/1, Relational Operator/1
  max/1 -> Relational Operator/2
  min/1 -> Relational Operator1/2
  AND/1 -> Switch/2
  Constant/1 -> Switch/3
  Relational Operator/1 -> AND/1
  Relational Operator1/1 -> AND/2
  Switch/1 -> Out1/1

== system gm_gauss_sobel_rgb_64bit_full/Subsystem/rgb_filter/Subsystem1/comparison1 ==
  In1 : Inport  OutDataTypeStr=uint8  PortDimensions=1  SampleTime=2.77039007092199e-06
  max : Inport  Port=2  OutDataTypeStr=uint8  PortDimensions=1  SampleTime=2.77039007092199e-06
  min : Inport  Port=3  OutDataTypeStr=uint8  PortDimensions=1  SampleTime=2.77039007092199e-06
  AND : Logic  IconShape=distinctive  AllPortsSameDT=off  OutDataTypeStr=boolean
  Constant : Constant  Value=0  OutDataTypeStr=uint8  SampleTime=-1
  Relational Operator : RelationalOperator  Operator=<=  OutDataTypeStr=boolean  RndMeth=Simplest  InputSameDT=off
  Relational Operator1 : RelationalOperator  OutDataTypeStr=boolean  RndMeth=Simplest  InputSameDT=off
  Switch : Switch  Criteria=u2 ~= 0  SaturateOnIntegerOverflow=off  InputSameDT=off
  Out1 : Outport  SampleTime=2.77039007092199e-06  InitialOutput=0
  wires:
  In1/1 -> Switch/1, Relational Operator1/1, Relational Operator/1
  max/1 -> Relational Operator/2
  min/1 -> Relational Operator1/2
  AND/1 -> Switch/2
  Constant/1 -> Switch/3
  Relational Operator/1 -> AND/1
  Relational Operator1/1 -> AND/2
  Switch/1 -> Out1/1

== system gm_gauss_sobel_rgb_64bit_full/Subsystem/rgb_filter/Subsystem1/comparison2 ==
  In1 : Inport  OutDataTypeStr=uint8  PortDimensions=1  SampleTime=2.77039007092199e-06
  max : Inport  Port=2  OutDataTypeStr=uint8  PortDimensions=1  SampleTime=2.77039007092199e-06
  min : Inport  Port=3  OutDataTypeStr=uint8  PortDimensions=1  SampleTime=2.77039007092199e-06
  AND : Logic  IconShape=distinctive  AllPortsSameDT=off  OutDataTypeStr=boolean
  Constant : Constant  Value=0  OutDataTypeStr=uint8  SampleTime=-1
  Relational Operator : RelationalOperator  Operator=<=  OutDataTypeStr=boolean  RndMeth=Simplest  InputSameDT=off
  Relational Operator1 : RelationalOperator  OutDataTypeStr=boolean  RndMeth=Simplest  InputSameDT=off
  Switch : Switch  Criteria=u2 ~= 0  SaturateOnIntegerOverflow=off  InputSameDT=off
  Out1 : Outport  SampleTime=2.77039007092199e-06  InitialOutput=0
  wires:
  In1/1 -> Switch/1, Relational Operator1/1, Relational Operator/1
  max/1 -> Relational Operator/2
  min/1 -> Relational Operator1/2
  AND/1 -> Switch/2
  Constant/1 -> Switch/3
  Relational Operator/1 -> AND/1
  Relational Operator1/1 -> AND/2
  Switch/1 -> Out1/1

== system gm_gauss_sobel_rgb_64bit_full/Subsystem/rgb_filter/Subsystem1/comparison3 ==
  In1 : Inport  OutDataTypeStr=uint8  PortDimensions=1  SampleTime=2.77039007092199e-06
  max : Inport  Port=2  OutDataTypeStr=uint8  PortDimensions=1  SampleTime=2.77039007092199e-06
  min : Inport  Port=3  OutDataTypeStr=uint8  PortDimensions=1  SampleTime=2.77039007092199e-06
  AND : Logic  IconShape=distinctive  AllPortsSameDT=off  OutDataTypeStr=boolean
  Constant : Constant  Value=0  OutDataTypeStr=uint8  SampleTime=-1
  Relational Operator : RelationalOperator  Operator=<=  OutDataTypeStr=boolean  RndMeth=Simplest  InputSameDT=off
  Relational Operator1 : RelationalOperator  OutDataTypeStr=boolean  RndMeth=Simplest  InputSameDT=off
  Switch : Switch  Criteria=u2 ~= 0  SaturateOnIntegerOverflow=off  InputSameDT=off
  Out1 : Outport  SampleTime=2.77039007092199e-06  InitialOutput=0
  wires:
  In1/1 -> Switch/1, Relational Operator1/1, Relational Operator/1
  max/1 -> Relational Operator/2
  min/1 -> Relational Operator1/2
  AND/1 -> Switch/2
  Constant/1 -> Switch/3
  Relational Operator/1 -> AND/1
  Relational Operator1/1 -> AND/2
  Switch/1 -> Out1/1

== system gm_gauss_sobel_rgb_64bit_full/Subsystem/rgb_filter/Subsystem1/comparison4 ==
  In1 : Inport  OutDataTypeStr=uint8  PortDimensions=1  SampleTime=2.77039007092199e-06
  max : Inport  Port=2  OutDataTypeStr=uint8  PortDimensions=1  SampleTime=2.77039007092199e-06
  min : Inport  Port=3  OutDataTypeStr=uint8  PortDimensions=1  SampleTime=2.77039007092199e-06
  AND : Logic  IconShape=distinctive  AllPortsSameDT=off  OutDataTypeStr=boolean
  Constant : Constant  Value=0  OutDataTypeStr=uint8  SampleTime=-1
  Relational Operator : RelationalOperator  Operator=<=  OutDataTypeStr=boolean  RndMeth=Simplest  InputSameDT=off
  Relational Operator1 : RelationalOperator  OutDataTypeStr=boolean  RndMeth=Simplest  InputSameDT=off
  Switch : Switch  Criteria=u2 ~= 0  SaturateOnIntegerOverflow=off  InputSameDT=off
  Out1 : Outport  SampleTime=2.77039007092199e-06  InitialOutput=0
  wires:
  In1/1 -> Switch/1, Relational Operator1/1, Relational Operator/1
  max/1 -> Relational Operator/2
  min/1 -> Relational Operator1/2
  AND/1 -> Switch/2
  Constant/1 -> Switch/3
  Relational Operator/1 -> AND/1
  Relational Operator1/1 -> AND/2
  Switch/1 -> Out1/1

== system gm_gauss_sobel_rgb_64bit_full/Subsystem/rgb_filter/Subsystem1/comparison6 ==
  In1 : Inport  OutDataTypeStr=uint8  PortDimensions=1  SampleTime=2.77039007092199e-06
  max : Inport  Port=2  OutDataTypeStr=uint8  PortDimensions=1  SampleTime=2.77039007092199e-06
  min : Inport  Port=3  OutDataTypeStr=uint8  PortDimensions=1  SampleTime=2.77039007092199e-06
  AND : Logic  IconShape=distinctive  AllPortsSameDT=off  OutDataTypeStr=boolean
  Constant : Constant  Value=0  OutDataTypeStr=uint8  SampleTime=-1
  Relational Operator : RelationalOperator  Operator=<=  OutDataTypeStr=boolean  RndMeth=Simplest  InputSameDT=off
  Relational Operator1 : RelationalOperator  OutDataTypeStr=boolean  RndMeth=Simplest  InputSameDT=off
  Switch : Switch  Criteria=u2 ~= 0  SaturateOnIntegerOverflow=off  InputSameDT=off
  Out1 : Outport  SampleTime=2.77039007092199e-06  InitialOutput=0
  wires:
  In1/1 -> Switch/1, Relational Operator1/1, Relational Operator/1
  max/1 -> Relational Operator/2
  min/1 -> Relational Operator1/2
  AND/1 -> Switch/2
  Constant/1 -> Switch/3
  Relational Operator/1 -> AND/1
  Relational Operator1/1 -> AND/2
  Switch/1 -> Out1/1

== system gm_gauss_sobel_rgb_64bit_full/Subsystem/conv_core_gauss/Subsystem1/slicer R operation1/Delay1 ==
  in0 : Inport  OutDataTypeStr=fixdt(0,8,0,'DataTypeOverride', 'Off')  SampleTime=2.77039007092199e-06
  <valid> : EnablePort  OutDataTypeStr=boolean
  Delay1 : Delay  DelayLength=double(1)  InitialCondition=0
  out0 : Outport  OutDataTypeStr=uint8  SampleTime=2.77039007092199e-06  InitialOutput=0
  wires:
  Delay1/1 -> out0/1
  in0/1 -> Delay1/1

== system gm_gauss_sobel_rgb_64bit_full/Subsystem/conv_core_gauss/Subsystem1/slicer R operation1/Delay2 ==
  in0 : Inport  OutDataTypeStr=fixdt(0,8,0,'DataTypeOverride', 'Off')  SampleTime=2.77039007092199e-06
  <valid> : EnablePort  OutDataTypeStr=boolean
  Delay2 : Delay  DelayLength=double(1)  InitialCondition=0
  out0 : Outport  OutDataTypeStr=uint8  SampleTime=2.77039007092199e-06  InitialOutput=0
  wires:
  Delay2/1 -> out0/1
  in0/1 -> Delay2/1

== system gm_gauss_sobel_rgb_64bit_full/Subsystem/conv_core_gauss/Subsystem1/slicer R operation1/Delay3 ==
  in0 : Inport  OutDataTypeStr=fixdt(0,8,0,'DataTypeOverride', 'Off')  SampleTime=2.77039007092199e-06
  <valid> : EnablePort  OutDataTypeStr=boolean
  Delay3 : Delay  DelayLength=double(1)  InitialCondition=0
  out0 : Outport  OutDataTypeStr=uint8  SampleTime=2.77039007092199e-06  InitialOutput=0
  wires:
  Delay3/1 -> out0/1
  in0/1 -> Delay3/1

== system gm_gauss_sobel_rgb_64bit_full/Subsystem/conv_core_gauss/Subsystem1/slicer R operation1/Delay4 ==
  in0 : Inport  OutDataTypeStr=fixdt(0,8,0,'DataTypeOverride', 'Off')  SampleTime=2.77039007092199e-06
  <valid> : EnablePort  OutDataTypeStr=boolean
  Delay4 : Delay  DelayLength=double(1)  InitialCondition=0
  out0 : Outport  OutDataTypeStr=uint8  SampleTime=2.77039007092199e-06  InitialOutput=0
  wires:
  Delay4/1 -> out0/1
  in0/1 -> Delay4/1

== system gm_gauss_sobel_rgb_64bit_full/Subsystem/conv_core_gauss/Subsystem1/slicer R operation1/Delay5 ==
  in0 : Inport  OutDataTypeStr=fixdt(0,8,0,'DataTypeOverride', 'Off')  SampleTime=2.77039007092199e-06
  <valid> : EnablePort  OutDataTypeStr=boolean
  Delay5 : Delay  DelayLength=double(1)  InitialCondition=0
  out0 : Outport  OutDataTypeStr=uint8  SampleTime=2.77039007092199e-06  InitialOutput=0
  wires:
  Delay5/1 -> out0/1
  in0/1 -> Delay5/1

== system gm_gauss_sobel_rgb_64bit_full/Subsystem/conv_core_gauss/Subsystem1/slicer R operation1/Delay6 ==
  in0 : Inport  OutDataTypeStr=fixdt(0,8,0,'DataTypeOverride', 'Off')  SampleTime=2.77039007092199e-06
  <valid> : EnablePort  OutDataTypeStr=boolean
  Delay6 : Delay  DelayLength=double(1)  InitialCondition=0
  out0 : Outport  OutDataTypeStr=uint8  SampleTime=2.77039007092199e-06  InitialOutput=0
  wires:
  Delay6/1 -> out0/1
  in0/1 -> Delay6/1

== system gm_gauss_sobel_rgb_64bit_full/Subsystem/conv_core_gauss/Subsystem1/slicer R operation1/Line buffer ==
  in0 : Inport  OutDataTypeStr=fixdt(0,8,0,'DataTypeOverride', 'Off')  SampleTime=2.77039007092199e-06
  <valid> : EnablePort  OutDataTypeStr=boolean
  Line buffer : Delay  DelayLength=double(750)  InitialCondition=0
  out0 : Outport  OutDataTypeStr=uint8  SampleTime=2.77039007092199e-06  InitialOutput=0
  wires:
  Line buffer/1 -> out0/1
  in0/1 -> Line buffer/1

== system gm_gauss_sobel_rgb_64bit_full/Subsystem/conv_core_gauss/Subsystem1/slicer R operation1/Line buffer1 ==
  in0 : Inport  OutDataTypeStr=fixdt(0,8,0,'DataTypeOverride', 'Off')  SampleTime=2.77039007092199e-06
  <valid> : EnablePort  OutDataTypeStr=boolean
  Line buffer1 : Delay  DelayLength=double(750)  InitialCondition=0
  out0 : Outport  OutDataTypeStr=uint8  SampleTime=2.77039007092199e-06  InitialOutput=0
  wires:
  Line buffer1/1 -> out0/1
  in0/1 -> Line buffer1/1

== system gm_gauss_sobel_rgb_64bit_full/Subsystem/conv_core_gauss/Subsystem1/slicer R operation2/Delay1 ==
  in0 : Inport  OutDataTypeStr=fixdt(0,8,0,'DataTypeOverride', 'Off')  SampleTime=2.77039007092199e-06
  <valid> : EnablePort  OutDataTypeStr=boolean
  Delay1 : Delay  DelayLength=double(1)  InitialCondition=0
  out0 : Outport  OutDataTypeStr=uint8  SampleTime=2.77039007092199e-06  InitialOutput=0
  wires:
  Delay1/1 -> out0/1
  in0/1 -> Delay1/1

== system gm_gauss_sobel_rgb_64bit_full/Subsystem/conv_core_gauss/Subsystem1/slicer R operation2/Delay2 ==
  in0 : Inport  OutDataTypeStr=fixdt(0,8,0,'DataTypeOverride', 'Off')  SampleTime=2.77039007092199e-06
  <valid> : EnablePort  OutDataTypeStr=boolean
  Delay2 : Delay  DelayLength=double(1)  InitialCondition=0
  out0 : Outport  OutDataTypeStr=uint8  SampleTime=2.77039007092199e-06  InitialOutput=0
  wires:
  Delay2/1 -> out0/1
  in0/1 -> Delay2/1

== system gm_gauss_sobel_rgb_64bit_full/Subsystem/conv_core_gauss/Subsystem1/slicer R operation2/Delay3 ==
  in0 : Inport  OutDataTypeStr=fixdt(0,8,0,'DataTypeOverride', 'Off')  SampleTime=2.77039007092199e-06
  <valid> : EnablePort  OutDataTypeStr=boolean
  Delay3 : Delay  DelayLength=double(1)  InitialCondition=0
  out0 : Outport  OutDataTypeStr=uint8  SampleTime=2.77039007092199e-06  InitialOutput=0
  wires:
  Delay3/1 -> out0/1
  in0/1 -> Delay3/1

== system gm_gauss_sobel_rgb_64bit_full/Subsystem/conv_core_gauss/Subsystem1/slicer R operation2/Delay4 ==
  in0 : Inport  OutDataTypeStr=fixdt(0,8,0,'DataTypeOverride', 'Off')  SampleTime=2.77039007092199e-06
  <valid> : EnablePort  OutDataTypeStr=boolean
  Delay4 : Delay  DelayLength=double(1)  InitialCondition=0
  out0 : Outport  OutDataTypeStr=uint8  SampleTime=2.77039007092199e-06  InitialOutput=0
  wires:
  Delay4/1 -> out0/1
  in0/1 -> Delay4/1

== system gm_gauss_sobel_rgb_64bit_full/Subsystem/conv_core_gauss/Subsystem1/slicer R operation2/Delay5 ==
  in0 : Inport  OutDataTypeStr=fixdt(0,8,0,'DataTypeOverride', 'Off')  SampleTime=2.77039007092199e-06
  <valid> : EnablePort  OutDataTypeStr=boolean
  Delay5 : Delay  DelayLength=double(1)  InitialCondition=0
  out0 : Outport  OutDataTypeStr=uint8  SampleTime=2.77039007092199e-06  InitialOutput=0
  wires:
  Delay5/1 -> out0/1
  in0/1 -> Delay5/1

== system gm_gauss_sobel_rgb_64bit_full/Subsystem/conv_core_gauss/Subsystem1/slicer R operation2/Delay6 ==
  in0 : Inport  OutDataTypeStr=fixdt(0,8,0,'DataTypeOverride', 'Off')  SampleTime=2.77039007092199e-06
  <valid> : EnablePort  OutDataTypeStr=boolean
  Delay6 : Delay  DelayLength=double(1)  InitialCondition=0
  out0 : Outport  OutDataTypeStr=uint8  SampleTime=2.77039007092199e-06  InitialOutput=0
  wires:
  Delay6/1 -> out0/1
  in0/1 -> Delay6/1

== system gm_gauss_sobel_rgb_64bit_full/Subsystem/conv_core_gauss/Subsystem1/slicer R operation2/Line buffer ==
  in0 : Inport  OutDataTypeStr=fixdt(0,8,0,'DataTypeOverride', 'Off')  SampleTime=2.77039007092199e-06
  <valid> : EnablePort  OutDataTypeStr=boolean
  Line buffer : Delay  DelayLength=double(750)  InitialCondition=0
  out0 : Outport  OutDataTypeStr=uint8  SampleTime=2.77039007092199e-06  InitialOutput=0
  wires:
  Line buffer/1 -> out0/1
  in0/1 -> Line buffer/1

== system gm_gauss_sobel_rgb_64bit_full/Subsystem/conv_core_gauss/Subsystem1/slicer R operation2/Line buffer1 ==
  in0 : Inport  OutDataTypeStr=fixdt(0,8,0,'DataTypeOverride', 'Off')  SampleTime=2.77039007092199e-06
  <valid> : EnablePort  OutDataTypeStr=boolean
  Line buffer1 : Delay  DelayLength=double(750)  InitialCondition=0
  out0 : Outport  OutDataTypeStr=uint8  SampleTime=2.77039007092199e-06  InitialOutput=0
  wires:
  Line buffer1/1 -> out0/1
  in0/1 -> Line buffer1/1

== system gm_gauss_sobel_rgb_64bit_full/Subsystem/conv_core_gauss/Subsystem1/slicer R operation3/Delay1 ==
  in0 : Inport  OutDataTypeStr=fixdt(0,8,0,'DataTypeOverride', 'Off')  SampleTime=2.77039007092199e-06
  <valid> : EnablePort  OutDataTypeStr=boolean
  Delay1 : Delay  DelayLength=double(1)  InitialCondition=0
  out0 : Outport  OutDataTypeStr=uint8  SampleTime=2.77039007092199e-06  InitialOutput=0
  wires:
  Delay1/1 -> out0/1
  in0/1 -> Delay1/1

== system gm_gauss_sobel_rgb_64bit_full/Subsystem/conv_core_gauss/Subsystem1/slicer R operation3/Delay2 ==
  in0 : Inport  OutDataTypeStr=fixdt(0,8,0,'DataTypeOverride', 'Off')  SampleTime=2.77039007092199e-06
  <valid> : EnablePort  OutDataTypeStr=boolean
  Delay2 : Delay  DelayLength=double(1)  InitialCondition=0
  out0 : Outport  OutDataTypeStr=uint8  SampleTime=2.77039007092199e-06  InitialOutput=0
  wires:
  Delay2/1 -> out0/1
  in0/1 -> Delay2/1

== system gm_gauss_sobel_rgb_64bit_full/Subsystem/conv_core_gauss/Subsystem1/slicer R operation3/Delay3 ==
  in0 : Inport  OutDataTypeStr=fixdt(0,8,0,'DataTypeOverride', 'Off')  SampleTime=2.77039007092199e-06
  <valid> : EnablePort  OutDataTypeStr=boolean
  Delay3 : Delay  DelayLength=double(1)  InitialCondition=0
  out0 : Outport  OutDataTypeStr=uint8  SampleTime=2.77039007092199e-06  InitialOutput=0
  wires:
  Delay3/1 -> out0/1
  in0/1 -> Delay3/1

== system gm_gauss_sobel_rgb_64bit_full/Subsystem/conv_core_gauss/Subsystem1/slicer R operation3/Delay4 ==
  in0 : Inport  OutDataTypeStr=fixdt(0,8,0,'DataTypeOverride', 'Off')  SampleTime=2.77039007092199e-06
  <valid> : EnablePort  OutDataTypeStr=boolean
  Delay4 : Delay  DelayLength=double(1)  InitialCondition=0
  out0 : Outport  OutDataTypeStr=uint8  SampleTime=2.77039007092199e-06  InitialOutput=0
  wires:
  Delay4/1 -> out0/1
  in0/1 -> Delay4/1

== system gm_gauss_sobel_rgb_64bit_full/Subsystem/conv_core_gauss/Subsystem1/slicer R operation3/Delay5 ==
  in0 : Inport  OutDataTypeStr=fixdt(0,8,0,'DataTypeOverride', 'Off')  SampleTime=2.77039007092199e-06
  <valid> : EnablePort  OutDataTypeStr=boolean
  Delay5 : Delay  DelayLength=double(1)  InitialCondition=0
  out0 : Outport  OutDataTypeStr=uint8  SampleTime=2.77039007092199e-06  InitialOutput=0
  wires:
  Delay5/1 -> out0/1
  in0/1 -> Delay5/1

== system gm_gauss_sobel_rgb_64bit_full/Subsystem/conv_core_gauss/Subsystem1/slicer R operation3/Delay6 ==
  in0 : Inport  OutDataTypeStr=fixdt(0,8,0,'DataTypeOverride', 'Off')  SampleTime=2.77039007092199e-06
  <valid> : EnablePort  OutDataTypeStr=boolean
  Delay6 : Delay  DelayLength=double(1)  InitialCondition=0
  out0 : Outport  OutDataTypeStr=uint8  SampleTime=2.77039007092199e-06  InitialOutput=0
  wires:
  Delay6/1 -> out0/1
  in0/1 -> Delay6/1

== system gm_gauss_sobel_rgb_64bit_full/Subsystem/conv_core_gauss/Subsystem1/slicer R operation3/Line buffer ==
  in0 : Inport  OutDataTypeStr=fixdt(0,8,0,'DataTypeOverride', 'Off')  SampleTime=2.77039007092199e-06
  <valid> : EnablePort  OutDataTypeStr=boolean
  Line buffer : Delay  DelayLength=double(750)  InitialCondition=0
  out0 : Outport  OutDataTypeStr=uint8  SampleTime=2.77039007092199e-06  InitialOutput=0
  wires:
  Line buffer/1 -> out0/1
  in0/1 -> Line buffer/1
